simulink model "setconfig_example_v21"  (R2017b)
settings: Solver=VariableStepAuto  StartTime=0.0  StopTime=20  RelTol=1e-3
libraries: simulink x1
settings Model: Creator=tmkhoyan  LastModifiedBy=tigran

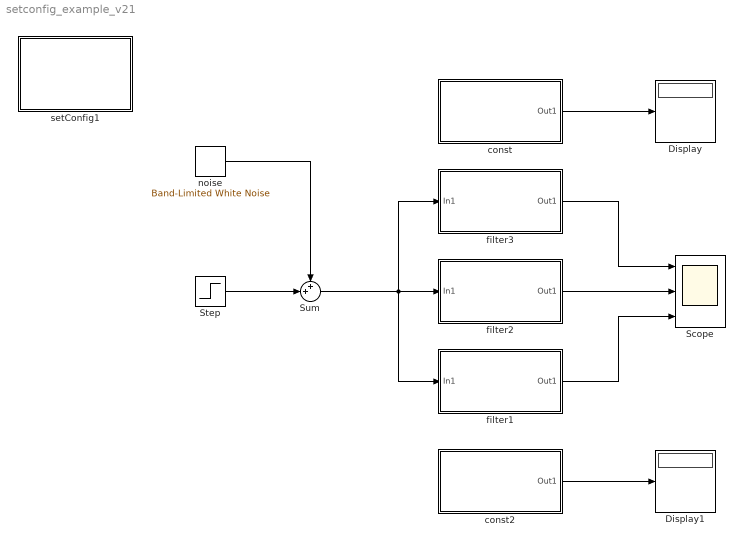
== system setconfig_example_v21 ==
  Display : Display
  Display1 : Display
  Scope : Scope  NumInputPorts=3
  Step : Step  SampleTime=0
  Sum : Sum  Inputs=++|
  const : Subsystem  mask{c1=0.01, c2=0.055, c3=0.026}
      mask prompts: c1 "constant 1"; c2 "constant 2"; c3 "constant 3"
  const2 : Subsystem  mask{k1=0.02, k2=100.005, k3=11.2}
      mask prompts: k1 "constant 1"; k2 "constant 2"; k3 "constant 3"
  filter1 : Subsystem
  filter2 : Subsystem
  filter3 : Subsystem
  noise : simulink/Sources/Band-Limited White Noise  Cov=0.02  Ts=0.0012  seed=[23341]
  setConfig1 : Subsystem  mask{filename='config/config_2.1.txt'}
      mask prompts: filename "config path"
      mask init:
      | setConfig(filename);
      mask DialogControl openfile Prompt: open file
      mask DialogControl openfile Callback:
      | flnm = [pwd(),'/',strip(get_param(gcb,'filename'),'''')];
      | try
      | open(flnm);
      | catch
      | warning('file %s not found',flnm);
      | end
      mask DialogControl setprm Prompt: Apply settings
      mask DialogControl setprm Callback:
      | flnm = strip(get_param(gcb,'filename'),'''');
      | try
      | setConfig(flnm);
      | catch
      | warning('file %s not found',flnm);
      | end
      mask Display: disp('x_o');
  wires:
  Sum/1 -> filter1/1(In1), filter2/1(In1), filter3/1(In1)
  filter2/1(Out1) -> Scope/2
  filter3/1(Out1) -> Scope/1
  filter1/1(Out1) -> Scope/3
  Step/1 -> Sum/2
  noise/1 -> Sum/1
  const/1(Out1) -> Display/1
  const2/1(Out1) -> Display1/1

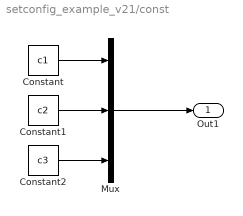
== system setconfig_example_v21/const ==
  Constant : Constant  Value=c1
  Constant1 : Constant  Value=c2
  Constant2 : Constant  Value=c3
  Mux : Mux  Inputs=3
  Out1 : Outport
  wires:
  Constant/1 -> Mux/1
  Constant1/1 -> Mux/2
  Constant2/1 -> Mux/3
  Mux/1 -> Out1/1

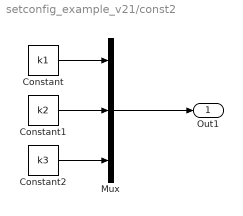
== system setconfig_example_v21/const2 ==
  Constant : Constant  Value=k1
  Constant1 : Constant  Value=k2
  Constant2 : Constant  Value=k3
  Mux : Mux  Inputs=3
  Out1 : Outport
  wires:
  Constant/1 -> Mux/1
  Constant1/1 -> Mux/2
  Constant2/1 -> Mux/3
  Mux/1 -> Out1/1

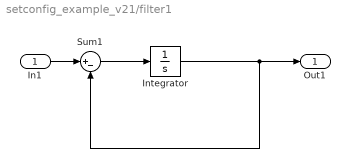
== system setconfig_example_v21/filter1 ==
  In1 : Inport
  Integrator : Integrator  InitialCondition=2
  Sum1 : Sum  Inputs=|+-
  Out1 : Outport
  wires:
  Sum1/1 -> Integrator/1
  Integrator/1 -> Out1/1, Sum1/2
  In1/1 -> Sum1/1

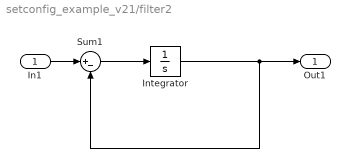
== system setconfig_example_v21/filter2 ==
  In1 : Inport
  Integrator : Integrator  InitialCondition=-2  UpperSaturationLimit=120
  Sum1 : Sum  Inputs=|+-
  Out1 : Outport
  wires:
  In1/1 -> Sum1/1
  Integrator/1 -> Sum1/2, Out1/1
  Sum1/1 -> Integrator/1

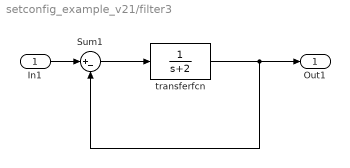
== system setconfig_example_v21/filter3 ==
  In1 : Inport
  Sum1 : Sum  Inputs=|+-
  transferfcn : TransferFcn  Denominator=[1 2]
  Out1 : Outport
  wires:
  Sum1/1 -> transferfcn/1
  transferfcn/1 -> Out1/1, Sum1/2
  In1/1 -> Sum1/1

== system setconfig_example_v21/setConfig1 ==
